simulink model "final_part5"  (R2023a)
settings: Solver=ode1  StartTime=0.0  StopTime=10.0  FixedStep=0.005  RelTol=1e-3
values from neighbouring files (symbols this model uses):
  a = 81.44    [DetermineTorqConstants.m]    (also in part4.m = 69.9384142006)
  A = [ 0 1 0 0 ... (first row only)    [part4.m]    (also in untitled2.m = [1;0])
  B = [ 0; -0.87; 0; 163]    [part4.m]
  C = [1 0 0 0 ; 0 0 1 0]    [part4.m]
undefined symbols (not defined in the file or in its folder): L
libraries: c6xlib x4, fricblocks x3
settings Model: Creator=rawnies2  LastModifiedBy=rawnies2
settings OptimizationCC: EnhancedBackFolding=on  PassReuseOutputArgsThreshold=0  OptimizeBlockOrder=speed  DifferentSizesBufferReuse=on  OptimizationCustomize=off
settings DebuggingCC: ParameterTunabilityLossMsg=error
settings HardwareCC: ProdBitPerInt=16  ProdBitPerPointer=16  ProdBitPerSizeT=16  ProdBitPerPtrDiffT=16  ProdLargestAtomicFloat=None  ProdWordSize=8  ProdHWDeviceType=Atmel->AVR  TargetBitPerPointer=64  TargetBitPerSizeT=64  TargetBitPerPtrDiffT=64  TargetLongLongMode=on  TargetIntDivRoundTo=Zero  TargetEndianess=LittleEndian  TargetWordSize=64  TargetHWDeviceType=MATLAB Host  ProdEqTarget=off
settings SFSimCC: MATLABDynamicMemAlloc=off
settings RTWCC: Description=Rapid Simulation Target  SystemTargetFile=rsim.tlc  TemplateMakefile=rsim_default_tmf  RTWVerbose=off
settings CodeAppCC: ForceParamTrailComments=on  OperatorAnnotations=on
settings RSimTargetCC: OptimizeReductions=off

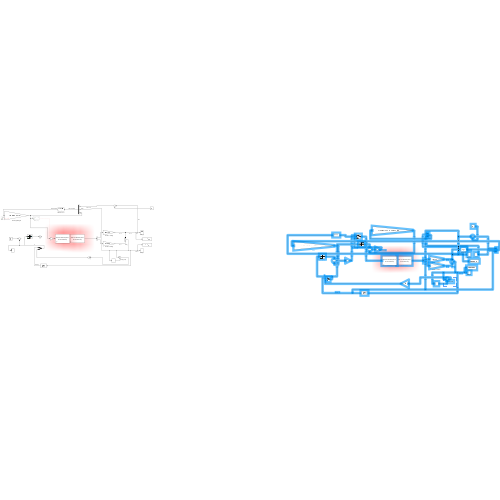
[thumbnail: Simulink's stored preview of the top-level diagram]
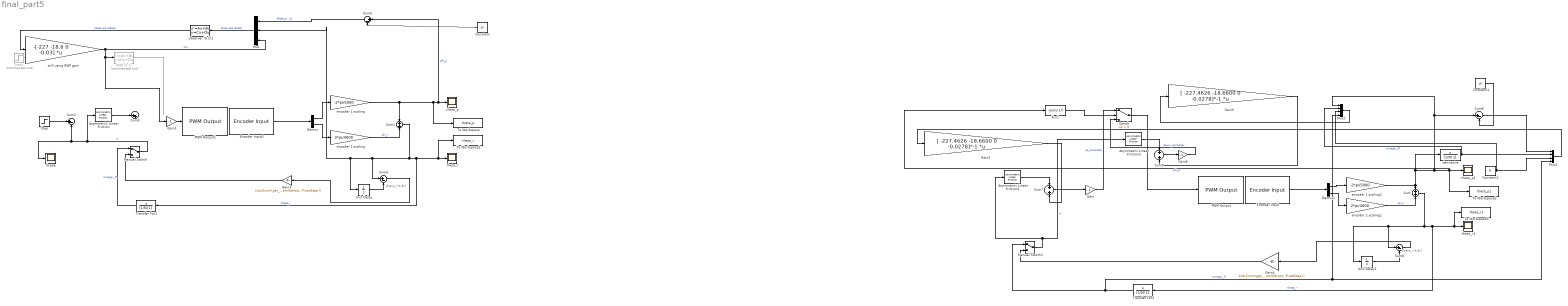
== system final_part5 ==
  note: theta_r(t-dt)
  note: theta_r(t-dt)
  Asymmetric Linear Friction : fricblocks/Asymmetric  Linear Friction  intercept1=0.6043  intercept2=-0.6143  slope1=0.01219  slope2=0.01291
  Asymmetric Linear Friction1 : fricblocks/Asymmetric  Linear Friction  intercept1=0.6043  intercept2=-0.6143  slope1=0.01219  slope2=0.01291
  Asymmetric Linear Friction2 : fricblocks/Asymmetric  Linear Friction  intercept1=0.6043  intercept2=-0.6143  slope1=0.01219  slope2=0.01291
  Constant : Constant  Value=pi
  Constant1 : Constant  Value=pi
  Constant2 : Constant  Value=0
  Demux : Demux  Outputs=2
  Demux1 : Demux  Outputs=2
  Encoder Input : c6xlib/Encoder Input  baseAddr=findParallelAddress  channels=[0 1]  sampleTime=str2num(get_param(bdroot, 'FixedStep'))
  Encoder Input1 : c6xlib/Encoder Input  baseAddr=findParallelAddress  channels=[0 1]  sampleTime=str2num(get_param(bdroot, 'FixedStep'))
  Fcn1 : Fcn  Expr=cos(u(1))
  Gain : Gain  Gain=-1
  Gain1 : Gain  Gain=-1
  Gain2 : Gain  Gain="[ -227.4626  -18.6600   0   -0.0278]*-1"  Multiplication=Matrix(K*u) (u vector)
  Gain3 : Gain  Gain=1/str2num(get_param(bdroot, 'FixedStep'))
  Gain4 : Gain  Gain=1/str2num(get_param(bdroot, 'FixedStep'))
  Gain5 : Gain  Gain="[ -227.4626  -18.6600   0   -0.0278]*-1"  Multiplication=Matrix(K*u) (u vector)
  Gain6 : Gain  Gain=-1
  Manual Switch : ManualSwitch
  Manual Switch1 : ManualSwitch
  Mux : Mux  Inputs=3
  Mux1 : Mux
  Mux2 : Mux
  PWM Output : c6xlib/PWM Output  baseAddr=findParallelAddress  channels=0  initialOutputs=0  finalOutputs=0  sampleTime=str2num(get_param(bdroot, 'FixedStep'))
  PWM Output1 : c6xlib/PWM Output  baseAddr=findParallelAddress  channels=0  initialOutputs=0  finalOutputs=0  sampleTime=str2num(get_param(bdroot, 'FixedStep'))
  RWP (4.1) : StateSpace  Commented=on  A="[ 0 1  ; a 0 ];"  B=[ 0; -0.87];  C=[ 0 0;0 0]  D=[ 0 ;0]  InitialCondition=0
  Scope : Scope
  Step : Step  Time=0  After=5  SampleTime=0
  Step2 : Step  Commented=on  Time=0  After=5  SampleTime=0
  Sum{,1,7,9} (4 alike) : Sum
  Sum{2,4..6,8} (5 alike) : Sum  Inputs=|+-
  Sum3 : Sum  Inputs=|++
  Switch : Switch  Criteria=u2 > Threshold  SaturateOnIntegerOverflow=off  InputSameDT=off
  To Workspace : ToWorkspace  VariableName=theta_p  SaveFormat=Structure With Time  SampleTime=-1
  To Workspace1 : ToWorkspace  VariableName=theta_r  SaveFormat=Structure With Time  SampleTime=-1
  To Workspace2 : ToWorkspace  VariableName=theta_p1  SaveFormat=Structure With Time  SampleTime=-1
  To Workspace3 : ToWorkspace  VariableName=theta_r1  SaveFormat=Structure With Time  SampleTime=-1
  Transfer Fcn1 : TransferFcn  Numerator=[1 0]  Denominator=[1/50 1]
  Transfer Fcn2 : TransferFcn  Numerator=[1 0]  Denominator=[1/50 1]
  Unit Delay : UnitDelay  SampleTime=-1  HasFrameUpgradeWarning=on
  Unit Delay1 : UnitDelay  SampleTime=-1  HasFrameUpgradeWarning=on
  derivative : TransferFcn  Numerator=[1 0]  Denominator=[1/50 1]
  encoder 1 scaling : Gain  Gain=-2*pi/5000
  encoder 1 scaling1 : Gain  Gain=-2*pi/5000
  encoder 2 scaling : Gain  Gain=2*pi/4000
  encoder 2 scaling1 : Gain  Gain=2*pi/4000
  observer (5.1)1 : StateSpace  A=A-L*C  B=[B L]  C=eye(4)  D=zeros(4, 3)  InitialCondition=0  ParameterTunability=Unconstrained
  still using RWP gain : Gain  Gain=-[-227 -18.6 0 -0.03]  Multiplication=Matrix(K*u) (u vector)
  theta_p : Scope
  theta_p1 : Scope
  theta_r : Scope
  theta_r1 : Scope
  wires:
  Unit Delay/1 -> Sum4/2
  Step/1 -> Sum2/1
  Gain1/1 -> PWM Output1/1
  Sum1/1 -> Mux/2, Unit Delay/1, Sum4/1, To Workspace1/1, theta_r/1, Transfer Fcn1/1  "theta_r"
  Demux/2 -> encoder 2 scaling/1
  Demux/1 -> encoder 1 scaling/1
  Manual Switch/1 -> Asymmetric Linear Friction/1, Scope/1, Sum2/2  "w"
  encoder 2 scaling/1 -> Sum1/2  "phi_r"
  Transfer Fcn1/1 -> Manual Switch/1  "omega _R"
  Gain3/1 -> Manual Switch/2
  Sum4/1 -> Gain3/1
  Encoder Input1/1 -> Demux/1
  Asymmetric Linear Friction/1 -> Sum3/1
  encoder 1 scaling/1 -> Sum1/1, To Workspace/1, Sum5/1, theta_p/1  "phi_p"
  still using RWP gain/1 -> RWP (4.1)/1, Gain1/1, Mux/3  "-Ku"
  Constant/1 -> Sum5/2
  Sum5/1 -> Mux/1  "theta_p - pi"
  Mux/1 -> observer (5.1)1/1  "observed states"
  Step2/1 -> ?
  RWP (4.1)/1 -> ?
  observer (5.1)1/1 -> still using RWP gain/1  "observed states"
  Switch/1 -> PWM Output/1
  Unit Delay1/1 -> Sum8/2
  derivative/1 -> Mux2/2, Mux1/2  "omega _R"
  Mux1/1 -> Gain2/1
  Sum6/1 -> Mux1/1
  Sum7/1 -> Gain/1
  Constant1/1 -> Sum6/2
  Asymmetric Linear Friction1/1 -> Sum7/1
  Gain2/1 -> Sum7/2
  Sum8/1 -> Gain4/1
  Gain/1 -> Switch/1  "up_controller"
  Constant2/1 -> Mux2/3, Mux1/3
  Sum/1 -> Sum8/1, Unit Delay1/1, Transfer Fcn2/1, To Workspace3/1, theta_r1/1  "theta_r"
  encoder 2 scaling1/1 -> Sum/2  "phi_r"
  Transfer Fcn2/1 -> Mux1/4, Mux2/4, Manual Switch1/1  "omega _R"
  Demux1/1 -> encoder 1 scaling1/1
  encoder 1 scaling1/1 -> Fcn1/1, To Workspace2/1, theta_p1/1, Mux2/1, Sum6/1, derivative/1, Sum/1  "phi_p"
  Demux1/2 -> encoder 2 scaling1/1
  Manual Switch1/1 -> Asymmetric Linear Friction2/1, Asymmetric Linear Friction1/1  "w"
  Encoder Input/1 -> Demux1/1
  Gain4/1 -> Manual Switch1/2
  Asymmetric Linear Friction2/1 -> Sum9/1
  Mux2/1 -> Gain5/1
  Sum9/1 -> Gain6/1
  Fcn1/1 -> Switch/2
  Gain6/1 -> Switch/3  "down_controller"
  Gain5/1 -> Sum9/2
